simulink model "servo"  (R2012a)
settings: Solver=ode45  StartTime=0.0  StopTime=2  RelTol=1e-3
InitFcn:
  | clear functions
libraries: truetime x1
settings Model: ExtModeTrigMode=oneshot  ExtModeArmWhenConnect=off  ExtModeAutoUpdateStatusClock=off  Creator=anton  LastModifiedBy=anton
settings DataIOCC: SaveFormat=Array  SignalLoggingSaveFormat=ModelDataLogs  ReturnWorkspaceOutputs=off  OutputTimes=[0.00199]
settings OptimizationCC: BlockReduction=off  BooleanDataType=off  ExpressionDepthLimit=2147483647  LifeSpan=inf  SimCompilerOptimization=Off
settings DebuggingCC: SaveWithParameterizedLinksMsg=none  UnderspecifiedInitializationDetection=Classic  MergeDetectMultiDrivingBlocksExec=none  SignalResolutionControl=TryResolveAllWithWarning  MultiTaskDSMMsg=warning  MultiTaskCondExecSysMsg=none  FcnCallInpInsideContextMsg=Enable All  StateNameClashWarn=warning  SFUnexpectedBacktrackingDiag=warning  SFNoUnconditionalDefaultTransitionDiag=warning
settings HardwareCC: ProdBitPerPointer=32  ProdLargestAtomicFloat=None  ProdIntDivRoundTo=Undefined  ProdEndianess=Unspecified  ProdWordSize=32  ProdHWDeviceType=32-bit Generic  TargetUnknown=on
settings ModelReferenceCC: PropagateSignalLabelsOutOfModel=off
settings SFSimCC: SimUseLocalCustomCode=off
settings RTWCC: RTWUseLocalCustomCode=off  RTWCompilerOptimization=Off
settings GRTTargetCC: CodeReplacementLibrary=C89/C90 (ANSI)  GeneratePreprocessorConditionals=Disable all  CombineOutputUpdateFcns=off  CPPClassGenCompliant=off  GRTInterface=on

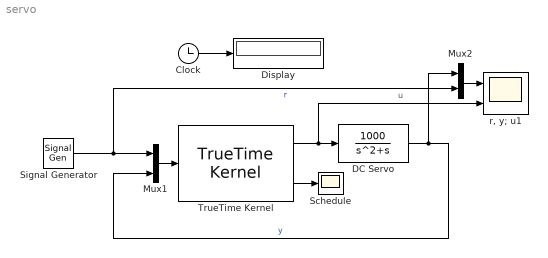
== system servo ==
  Clock : Clock
  DC Servo : TransferFcn  Numerator=[1000]  Denominator=[1 1 0]
  Display : Display
  Mux1 : Mux  Inputs=2
  Mux2 : Mux  Inputs=2
  Schedule : Scope
      settings: TimeRange=2  TickLabels=on  MaxDataPoints=5000  SaveToWorkspace=off  SaveName=ScopeData2  YMin=0.8  YMax=1.7  SampleTime=-1  DataFormat=Array
  Signal Generator : SignalGenerator  WaveForm=square
  TrueTime Kernel : truetime/TrueTime Kernel  sfun=servo_init_new  args=4  ninputsoutputs=[2 1]  ntriggers=0  trigtype=falling  nwnodenbr=[]  clockoffsetdrift=[0 0]  schedoutput=on  battery=off  poweroutput=off
  "r, y; u1" : Scope  NumInputPorts=2
      settings: TimeRange=1  MaxDataPoints=5000  SaveToWorkspace=off  SaveName=y  YMin=-1.5~-4  YMax=1.5~4  SampleTime=-1
  wires:
  TrueTime Kernel/1 -> DC Servo/1, "r, y; u1"/2  "u"
  Signal Generator/1 -> Mux1/1, Mux2/2  "r"
  Clock/1 -> Display/1
  DC Servo/1 -> Mux1/2, Mux2/1  "y"
  Mux1/1 -> TrueTime Kernel/1
  TrueTime Kernel/2 -> Schedule/1
  Mux2/1 -> "r, y; u1"/1
